simulink model "Model_Building_Method"  (R2024b)
settings: Solver=VariableStepAuto  StartTime=0.0  StopTime=20  RelTol=1e-3
settings Model: Creator=User  LastModifiedBy=User

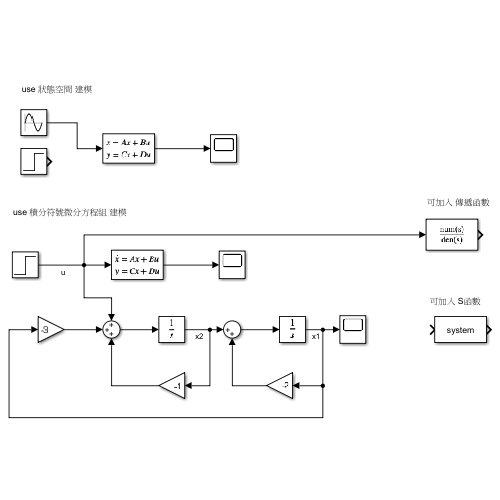
[thumbnail: Simulink's stored preview of the top-level diagram]
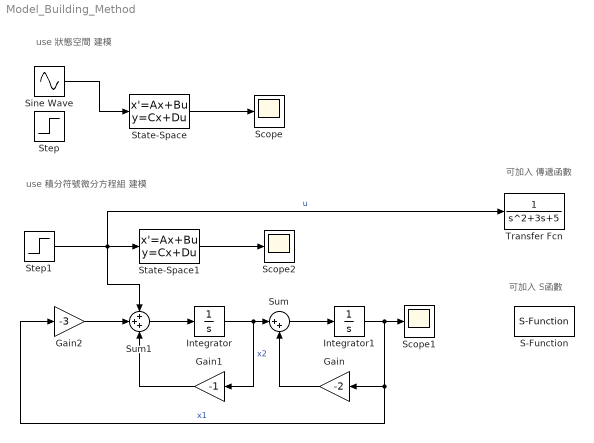
== system Model_Building_Method ==
  note: use 積分符號微分方程組 建模
  note: use 狀態空間 建模
  note: 可加入 傳遞函數
  note: 可加入 S函數
  Gain : Gain  Gain=-2
  Gain1 : Gain  Gain=-1
  Gain2 : Gain  Gain=-3
  Integrator : Integrator  InitialCondition=1
  Integrator1 : Integrator  InitialCondition=2
  S-Function : S-Function  SFunctionDeploymentMode=off  EnableBusSupport=off
  Scope : Scope
  Scope1 : Scope
  Scope2 : Scope
  Sine Wave : Sin  SampleTime=0
  State-Space : StateSpace  A=[-2, 1;-3,-1]  B=[0;1]  C=[1,0]  D=0  InitialCondition=[1,2]
  State-Space1 : StateSpace  A=[-2, 1;-3,-1]  B=[0;1]  C=[1,0]  D=0  InitialCondition=[1,2]
  Step : Step  SampleTime=0
  Step1 : Step  SampleTime=0
  Sum : Sum  Inputs=|++
  Sum1 : Sum  Inputs=+++
  Transfer Fcn : TransferFcn  Denominator=[1 3 5]
  wires:
  Sine Wave/1 -> State-Space/1
  State-Space/1 -> Scope/1
  Sum/1 -> Integrator1/1
  Integrator1/1 -> Gain/1, Gain2/1, Scope1/1  "x1"
  Gain/1 -> Sum/2
  Integrator/1 -> Gain1/1, Sum/1  "x2"
  Sum1/1 -> Integrator/1
  State-Space1/1 -> Scope2/1
  Step1/1 -> Transfer Fcn/1, Sum1/1, State-Space1/1  "u"
  Gain1/1 -> Sum1/3
  Gain2/1 -> Sum1/2
